simulink model "fiveleveldiode"  (Simulink 7.3)
settings: Solver=ode45  StartTime=0.0  StopTime=0.1  RelTol=1e-3
InitFcn:
  | clear;
  | clc;
  | f=50;
  | fs=4000;
libraries: powerlib x56, simulink x12, powerlib_extras x3
Description:
  | This model includes five level three phase diode clamped bridge. The control is implemented
  | using the multi carrier sinosoidal PWM technique.
  | 
  | This was created by Syed Abdul Rahman Kashif
  | University of Paderborn
  | Germany
settings Model: Creator=Kashif  LastModifiedBy=Sravani Harshini

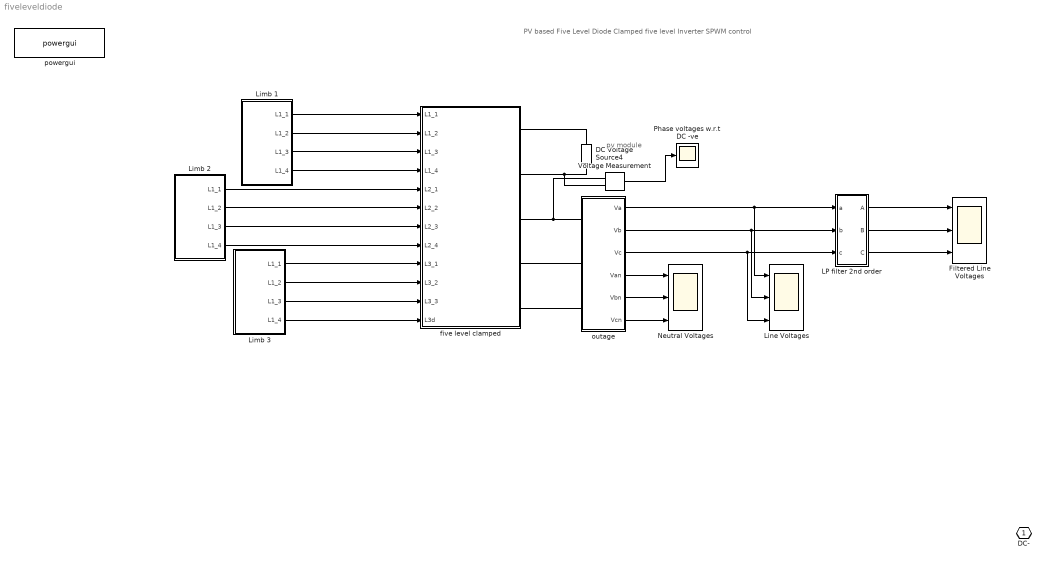
== system fiveleveldiode ==
  note: PV based Five Level Diode Clamped five level Inverter SPWM control
  note: pv module
  DC Voltage Source4 : powerlib/Electrical Sources/DC Voltage Source  DialogController=POWERSYS.PowerSysDialog  SystemSampleTime=-1  Amplitude=400  Measurements=None
  Filtered Line Voltages : Scope  NumInputPorts=3
      settings: YMin=-45~-35~-45  YMax=70~70~70  SaveName=Filtered_Line_Voltages  MaxDataPoints=5000000  SampleInput=on  SampleTime=5e-6
  LP filter 2nd order : Subsystem  mask{cutoff_frequency=500, damping_factor=0.707}
      mask prompts: cutoff_frequency "Cut off frequency"; damping_factor "Damping Factor"
  Limb 1 : Subsystem
  Limb 2 : Subsystem
  Limb 3 : Subsystem
  Line Voltages : Scope  NumInputPorts=3
      settings: YMin=-45~-35~-45  YMax=70~70~70  SaveName=Line_voltages  MaxDataPoints=5000000  SampleInput=on  SampleTime=5e-6
  Neutral Voltages : Scope  NumInputPorts=3
      settings: YMin=-45~-35~-45  YMax=70~70~70  SaveName=Neutral_voltages  MaxDataPoints=5000000  SampleInput=on  SampleTime=5e-6
  Phase voltages w.r.t DC -ve : Scope
      settings: YMin=0  YMax=100  SaveName=Phase_voltage_DC0  MaxDataPoints=5000000  SampleInput=on  SampleTime=5e-6
  Voltage Measurement : powerlib/Measurements/Voltage Measurement  DialogController=POWERSYS.PowerSysDialog  SystemSampleTime=-1  PhasorSimulation=off  OutputType=Complex  PSBequivalent=0
  five level clamped : Subsystem
      mask Description:
      | This includes five level three phase diode clamped bridge.
      | This was created by Syed Abdul Rahman Kashif
      | University of Paderborn
      | Germany
  outage : Subsystem
  powergui : powerlib/powergui  Priority=1  SystemSampleTime=-1  SimulationMode=Discrete  SampleTime=2e-6  frequency=60  SPID=off  DisableSnubberDevices=off  DisableRonSwitches=off  DisableVfSwitches=off  SwTol=0  Interpol=off  frequencyindice=0  echomessages=off  HookPort=off  DisplayEquations=off  FunctionMessages=off  EnableUseOfTLC=off  x0status=blocks  RestoreLinks=warning  Frange=[0:2:500]  Ylog=off  Xlog=on  ShowGrid=off  save=off  variable=ZData  structure=Filtered_Line_Voltages  ZoomFFT=off  StartTime=0.04  cycles=1  DisplayStyle=2  fundamental=50  FreqAxis=off  MaxFrequency=10000  frequencyindicesteady=1  RmsSteady=1  display=off  Ts=0  methode=off
  DC- : PMIOPort  Port=1  Side=Left
  wires:
  Limb 1/1(L1_1) -> five level clamped/1(L1_1)
  Limb 1/2(L1_2) -> five level clamped/2(L1_2)
  Limb 1/3(L1_3) -> five level clamped/3(L1_3)
  Limb 1/4(L1_4) -> five level clamped/4(L1_4)
  outage/4(Van) -> Neutral Voltages/1
  outage/5(Vbn) -> Neutral Voltages/2
  outage/6(Vcn) -> Neutral Voltages/3
  Voltage Measurement/1 -> Phase voltages w.r.t DC -ve/1
  Limb 2/1(L1_1) -> five level clamped/5(L2_1)
  Limb 2/2(L1_2) -> five level clamped/6(L2_2)
  Limb 2/3(L1_3) -> five level clamped/7(L2_3)
  Limb 2/4(L1_4) -> five level clamped/8(L2_4)
  Limb 3/1(L1_1) -> five level clamped/9(L3_1)
  Limb 3/2(L1_2) -> five level clamped/10(L3_2)
  Limb 3/3(L1_3) -> five level clamped/11(L3_3)
  Limb 3/4(L1_4) -> five level clamped/12(L3d)
  outage/1(Va) -> LP filter 2nd order/1(a), Line Voltages/1
  outage/2(Vb) -> LP filter 2nd order/2(b), Line Voltages/2
  outage/3(Vc) -> LP filter 2nd order/3(c), Line Voltages/3
  LP filter 2nd order/1(A) -> Filtered Line Voltages/1
  LP filter 2nd order/2(B) -> Filtered Line Voltages/2
  LP filter 2nd order/3(C) -> Filtered Line Voltages/3
  connections:
  five level clamped/RConn2 -- DC Voltage Source4/LConn1 -- Voltage Measurement/LConn2
  five level clamped/RConn1 -- DC Voltage Source4/RConn1
  five level clamped/RConn5 -- outage/LConn3
  five level clamped/RConn4 -- outage/LConn2
  five level clamped/RConn3 -- outage/LConn1 -- Voltage Measurement/LConn1

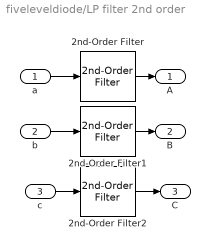
== system fiveleveldiode/LP filter 2nd order ==
  a : Inport  OutDataType=sfix(16)  OutScaling=2^0
  b : Inport  Port=2  OutDataType=sfix(16)  OutScaling=2^0
  c : Inport  Port=3  OutDataType=sfix(16)  OutScaling=2^0
  2nd-Order Filter : powerlib_extras/Control  Blocks/2nd-Order Filter  DialogController=POWERSYS.PowerSysDialog  SystemSampleTime=-1  FilterType=Lowpass  Fo=cutoff_frequency  Zeta=damping_factor  Initialize=off  Vac_Init=[1 45 60]  Vdc_Init=-0.5  PlotResponse=off  param1=[1 500 1]
  2nd-Order Filter1 : powerlib_extras/Control  Blocks/2nd-Order Filter  DialogController=POWERSYS.PowerSysDialog  SystemSampleTime=-1  FilterType=Lowpass  Fo=cutoff_frequency  Zeta=damping_factor  Initialize=off  Vac_Init=[1 45 60]  Vdc_Init=-0.5  PlotResponse=off  param1=[1 500 1]
  2nd-Order Filter2 : powerlib_extras/Control  Blocks/2nd-Order Filter  DialogController=POWERSYS.PowerSysDialog  SystemSampleTime=-1  FilterType=Lowpass  Fo=cutoff_frequency  Zeta=damping_factor  Initialize=off  Vac_Init=[1 45 60]  Vdc_Init=-0.5  PlotResponse=off  param1=[1 500 1]
  A : Outport  OutDataType=sfix(16)  OutScaling=2^0
  B : Outport  Port=2  OutDataType=sfix(16)  OutScaling=2^0
  C : Outport  Port=3  OutDataType=sfix(16)  OutScaling=2^0
  wires:
  a/1 -> 2nd-Order Filter/1
  2nd-Order Filter/1 -> A/1
  b/1 -> 2nd-Order Filter1/1
  2nd-Order Filter1/1 -> B/1
  c/1 -> 2nd-Order Filter2/1
  2nd-Order Filter2/1 -> C/1

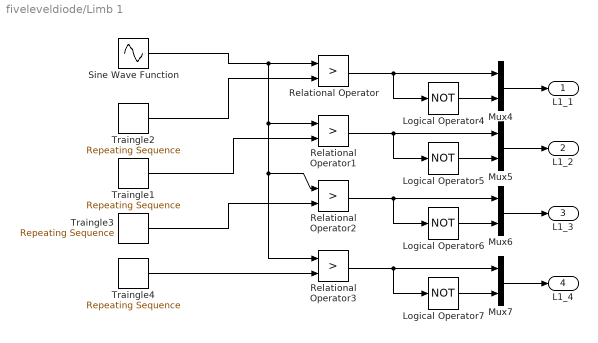
== system fiveleveldiode/Limb 1 ==
  Logical Operator{4..7} (4 alike) : Logic  Operator=NOT  AllPortsSameDT=off  OutDataTypeMode=boolean  OutDataTypeStr=boolean
  Mux{4..7} (4 alike) : Mux  Inputs=2
  Relational Operator{,1..3} (4 alike) : RelationalOperator  Operator=>  LogicOutDataTypeMode=boolean  LogicDataType=fixdt(0, 8)  OutDataTypeStr=boolean
  Sine Wave Function : Sin  Amplitude=5  Bias=5  Frequency=f*2*pi  Phase=0  Samples=10  SampleTime=0  Offset=0
  Traingle1 : simulink/Sources/Repeating Sequence  SystemSampleTime=-1  rep_seq_t=[0 1/fs]  rep_seq_y=[5 7.5]
  Traingle2 : simulink/Sources/Repeating Sequence  SystemSampleTime=-1  rep_seq_t=[0 1/fs]  rep_seq_y=[7.5 10]
  Traingle3 : simulink/Sources/Repeating Sequence  SystemSampleTime=-1  rep_seq_t=[0 1/fs]  rep_seq_y=[2.5 5]
  Traingle4 : simulink/Sources/Repeating Sequence  SystemSampleTime=-1  rep_seq_t=[0 1/fs]  rep_seq_y=[0 2.5]
  L1_1 : Outport  OutDataType=sfix(16)  OutScaling=2^0
  L1_2 : Outport  Port=2  OutDataType=sfix(16)  OutScaling=2^0
  L1_3 : Outport  Port=3  OutDataType=sfix(16)  OutScaling=2^0
  L1_4 : Outport  Port=4  OutDataType=sfix(16)  OutScaling=2^0
  wires:
  Sine Wave Function/1 -> Relational Operator/1, Relational Operator1/1, Relational Operator2/1, Relational Operator3/1
  Traingle2/1 -> Relational Operator/2
  Traingle4/1 -> Relational Operator3/2
  Traingle3/1 -> Relational Operator2/2
  Traingle1/1 -> Relational Operator1/2
  Relational Operator/1 -> Logical Operator4/1, Mux4/1
  Logical Operator4/1 -> Mux4/2
  Mux4/1 -> L1_1/1
  Relational Operator1/1 -> Mux5/1, Logical Operator5/1
  Logical Operator5/1 -> Mux5/2
  Mux5/1 -> L1_2/1
  Relational Operator2/1 -> Logical Operator6/1, Mux6/1
  Logical Operator6/1 -> Mux6/2
  Mux6/1 -> L1_3/1
  Relational Operator3/1 -> Mux7/1, Logical Operator7/1
  Logical Operator7/1 -> Mux7/2
  Mux7/1 -> L1_4/1

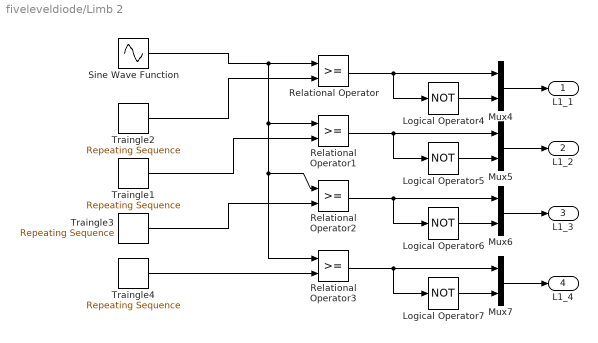
== system fiveleveldiode/Limb 2 ==
  Logical Operator{4..7} (4 alike) : Logic  Operator=NOT  AllPortsSameDT=off  OutDataTypeMode=boolean  OutDataTypeStr=boolean
  Mux{4..7} (4 alike) : Mux  Inputs=2
  Relational Operator{,1..3} (4 alike) : RelationalOperator  LogicOutDataTypeMode=boolean  LogicDataType=fixdt(0, 8)  OutDataTypeStr=boolean
  Sine Wave Function : Sin  Amplitude=5  Bias=5  Frequency=f*2*pi  Phase=4*pi/3  Samples=10  SampleTime=0  Offset=0
  Traingle1 : simulink/Sources/Repeating Sequence  SystemSampleTime=-1  rep_seq_t=[0 1/fs]  rep_seq_y=[5 7.5]
  Traingle2 : simulink/Sources/Repeating Sequence  SystemSampleTime=-1  rep_seq_t=[0 1/fs]  rep_seq_y=[7.5 10]
  Traingle3 : simulink/Sources/Repeating Sequence  SystemSampleTime=-1  rep_seq_t=[0 1/fs]  rep_seq_y=[2.5 5]
  Traingle4 : simulink/Sources/Repeating Sequence  SystemSampleTime=-1  rep_seq_t=[0 1/fs]  rep_seq_y=[0 2.5]
  L1_1 : Outport  OutDataType=sfix(16)  OutScaling=2^0
  L1_2 : Outport  Port=2  OutDataType=sfix(16)  OutScaling=2^0
  L1_3 : Outport  Port=3  OutDataType=sfix(16)  OutScaling=2^0
  L1_4 : Outport  Port=4  OutDataType=sfix(16)  OutScaling=2^0
  wires:
  Mux7/1 -> L1_4/1
  Logical Operator7/1 -> Mux7/2
  Relational Operator3/1 -> Logical Operator7/1, Mux7/1
  Mux6/1 -> L1_3/1
  Logical Operator6/1 -> Mux6/2
  Relational Operator2/1 -> Mux6/1, Logical Operator6/1
  Mux5/1 -> L1_2/1
  Logical Operator5/1 -> Mux5/2
  Relational Operator1/1 -> Logical Operator5/1, Mux5/1
  Mux4/1 -> L1_1/1
  Logical Operator4/1 -> Mux4/2
  Relational Operator/1 -> Mux4/1, Logical Operator4/1
  Traingle1/1 -> Relational Operator1/2
  Traingle3/1 -> Relational Operator2/2
  Traingle4/1 -> Relational Operator3/2
  Traingle2/1 -> Relational Operator/2
  Sine Wave Function/1 -> Relational Operator3/1, Relational Operator2/1, Relational Operator1/1, Relational Operator/1

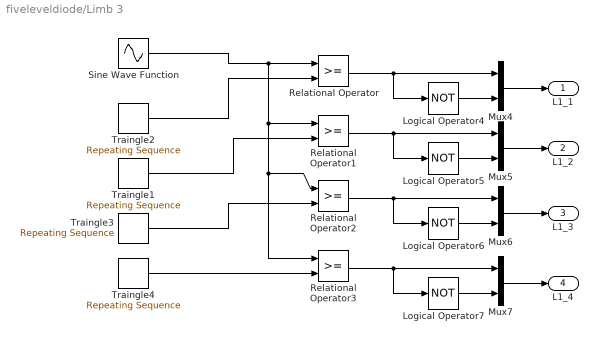
== system fiveleveldiode/Limb 3 ==
  Logical Operator{4..7} (4 alike) : Logic  Operator=NOT  AllPortsSameDT=off  OutDataTypeMode=boolean  OutDataTypeStr=boolean
  Mux{4..7} (4 alike) : Mux  Inputs=2
  Relational Operator{,1..3} (4 alike) : RelationalOperator  LogicOutDataTypeMode=boolean  LogicDataType=fixdt(0, 8)  OutDataTypeStr=boolean
  Sine Wave Function : Sin  Amplitude=5  Bias=5  Frequency=f*2*pi  Phase=2*pi/3  Samples=10  SampleTime=0  Offset=0
  Traingle1 : simulink/Sources/Repeating Sequence  SystemSampleTime=-1  rep_seq_t=[0 1/fs]  rep_seq_y=[5 7.5]
  Traingle2 : simulink/Sources/Repeating Sequence  SystemSampleTime=-1  rep_seq_t=[0 1/fs]  rep_seq_y=[7.5 10]
  Traingle3 : simulink/Sources/Repeating Sequence  SystemSampleTime=-1  rep_seq_t=[0 1/fs]  rep_seq_y=[2.5 5]
  Traingle4 : simulink/Sources/Repeating Sequence  SystemSampleTime=-1  rep_seq_t=[0 1/fs]  rep_seq_y=[0 2.5]
  L1_1 : Outport  OutDataType=sfix(16)  OutScaling=2^0
  L1_2 : Outport  Port=2  OutDataType=sfix(16)  OutScaling=2^0
  L1_3 : Outport  Port=3  OutDataType=sfix(16)  OutScaling=2^0
  L1_4 : Outport  Port=4  OutDataType=sfix(16)  OutScaling=2^0
  wires:
  Sine Wave Function/1 -> Relational Operator/1, Relational Operator1/1, Relational Operator2/1, Relational Operator3/1
  Traingle2/1 -> Relational Operator/2
  Traingle4/1 -> Relational Operator3/2
  Traingle3/1 -> Relational Operator2/2
  Traingle1/1 -> Relational Operator1/2
  Relational Operator/1 -> Logical Operator4/1, Mux4/1
  Logical Operator4/1 -> Mux4/2
  Mux4/1 -> L1_1/1
  Relational Operator1/1 -> Mux5/1, Logical Operator5/1
  Logical Operator5/1 -> Mux5/2
  Mux5/1 -> L1_2/1
  Relational Operator2/1 -> Logical Operator6/1, Mux6/1
  Logical Operator6/1 -> Mux6/2
  Mux6/1 -> L1_3/1
  Relational Operator3/1 -> Mux7/1, Logical Operator7/1
  Logical Operator7/1 -> Mux7/2
  Mux7/1 -> L1_4/1

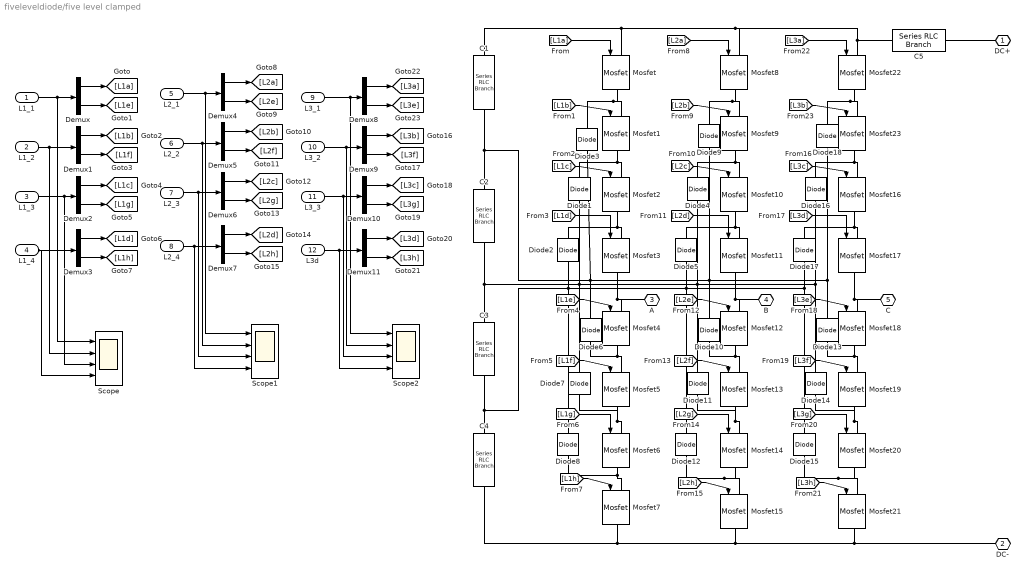
== system fiveleveldiode/five level clamped ==
  L1_1 : Inport  OutDataType=fixdt(1, 16)  OutScaling=2^0
  L1_2 : Inport  Port=2  OutDataType=fixdt(1, 16)  OutScaling=2^0
  L1_3 : Inport  Port=3  OutDataType=fixdt(1, 16)  OutScaling=2^0
  L1_4 : Inport  Port=4  OutDataType=fixdt(1, 16)  OutScaling=2^0
  L2_1 : Inport  Port=5  OutDataType=fixdt(1, 16)  OutScaling=2^0
  L2_2 : Inport  Port=6  OutDataType=fixdt(1, 16)  OutScaling=2^0
  L2_3 : Inport  Port=7  OutDataType=fixdt(1, 16)  OutScaling=2^0
  L2_4 : Inport  Port=8  OutDataType=fixdt(1, 16)  OutScaling=2^0
  L3_1 : Inport  Port=9  OutDataType=fixdt(1, 16)  OutScaling=2^0
  L3_2 : Inport  Port=10  OutDataType=fixdt(1, 16)  OutScaling=2^0
  L3_3 : Inport  Port=11  OutDataType=fixdt(1, 16)  OutScaling=2^0
  L3d : Inport  Port=12  OutDataType=fixdt(1, 16)  OutScaling=2^0
  C{1..4} (4 alike) : powerlib/Elements/Series RLC Branch  DialogController=POWERSYS.PowerSysDialog  PhysicalDomain=powersysdomain  SubClassName=unknown  LeftPortType=p1  RightPortType=p1  LConnTagsString=__new0  RConnTagsString=__new0  BranchType=C  Resistance=1  Inductance=1.0  SetiL0=off  InitialCurrent=0  Capacitance=2200e-6  Setx0=off  InitialVoltage=0  Measurements=None
  C5 : powerlib/Elements/Series RLC Branch  DialogController=POWERSYS.PowerSysDialog  PhysicalDomain=powersysdomain  SubClassName=unknown  LeftPortType=p1  RightPortType=p1  LConnTagsString=__new0  RConnTagsString=__new0  BranchType=R  Resistance=1  Inductance=1.0  SetiL0=off  InitialCurrent=0  Capacitance=2200e-6  Setx0=off  InitialVoltage=0  Measurements=None
  Demux{,1..11} (12 alike) : Demux  Outputs=2
  Diode{1..18} (18 alike) : powerlib/Power Electronics/Diode  DialogController=POWERSYS.PowerSysDialog  SystemSampleTime=-1  Ron=0.001  Lon=0  Vf=0.8  IC=0  UseSnubber=off  Rs=500  Cs=250e-9  Measurements=off
  Mosfet{,1..23} (24 alike) : powerlib/Power Electronics/Mosfet  DialogController=POWERSYS.PowerSysDialog  SystemSampleTime=-1  Ron=0.1  Lon=0  Rd=0.01  Vfd=0  IC=0  Rs=1e5  Cs=inf  Measurements=off
  Scope : Scope  NumInputPorts=4
      settings: YMin=-5~-5~-5~-5  YMax=5~5~5~5  MaxDataPoints=5000000
  Scope1 : Scope  NumInputPorts=4
      settings: YMin=-5~-5~-5~-5  YMax=5~5~5~5  SaveName=ScopeData2  MaxDataPoints=5000000
  Scope2 : Scope  NumInputPorts=4
      settings: YMin=-5~-5~-5~-5  YMax=5~5~5~5  SaveName=ScopeData3  MaxDataPoints=5000000
  DC+ : PMIOPort  Port=1  Side=Right
  DC- : PMIOPort  Port=2  Side=Right
  A : PMIOPort  Port=3  Side=Right
  B : PMIOPort  Port=4  Side=Right
  C : PMIOPort  Port=5  Side=Right
  wires:
  Demux/1 -> [L1a]
  Demux/2 -> [L1e]
  Demux1/1 -> [L1b]
  Demux1/2 -> [L1f]
  Demux2/1 -> [L1c]
  Demux2/2 -> [L1g]
  Demux3/1 -> [L1d]
  Demux3/2 -> [L1h]
  L1_1/1 -> Demux/1, Scope/1
  L1_2/1 -> Demux1/1, Scope/2
  L1_3/1 -> Demux2/1, Scope/3
  L1_4/1 -> Demux3/1, Scope/4
  Demux4/1 -> [L2a]
  Demux4/2 -> [L2e]
  Demux5/1 -> [L2b]
  Demux5/2 -> [L2f]
  Demux6/1 -> [L2c]
  Demux6/2 -> [L2g]
  Demux7/1 -> [L2d]
  Demux7/2 -> [L2h]
  L2_1/1 -> Demux4/1, Scope1/1
  L2_2/1 -> Demux5/1, Scope1/2
  L2_3/1 -> Demux6/1, Scope1/3
  L2_4/1 -> Demux7/1, Scope1/4
  Demux8/1 -> [L3a]
  Demux8/2 -> [L3e]
  Demux9/1 -> [L3b]
  Demux9/2 -> [L3f]
  Demux10/1 -> [L3c]
  Demux10/2 -> [L3g]
  Demux11/1 -> [L3d]
  Demux11/2 -> [L3h]
  L3_1/1 -> Demux8/1, Scope2/1
  L3_2/1 -> Demux9/1, Scope2/2
  L3_3/1 -> Demux10/1, Scope2/3
  L3d/1 -> Demux11/1, Scope2/4
  [L1a] -> Mosfet/1
  [L1b] -> Mosfet1/1
  [L1c] -> Mosfet2/1
  [L1d] -> Mosfet3/1
  [L1e] -> Mosfet4/1
  [L1f] -> Mosfet5/1
  [L1g] -> Mosfet6/1
  [L1h] -> Mosfet7/1
  [L2a] -> Mosfet8/1
  [L2b] -> Mosfet9/1
  [L2c] -> Mosfet10/1
  [L2d] -> Mosfet11/1
  [L2e] -> Mosfet12/1
  [L2f] -> Mosfet13/1
  [L2g] -> Mosfet14/1
  [L2h] -> Mosfet15/1
  [L3a] -> Mosfet22/1
  [L3b] -> Mosfet23/1
  [L3c] -> Mosfet16/1
  [L3d] -> Mosfet17/1
  [L3e] -> Mosfet18/1
  [L3f] -> Mosfet19/1
  [L3g] -> Mosfet20/1
  [L3h] -> Mosfet21/1
  connections:
  Diode3/RConn1 -- Mosfet1/LConn1 -- Mosfet/RConn1
  Mosfet1/RConn1 -- Mosfet2/LConn1 -- Diode1/RConn1
  Mosfet3/RConn1 -- Mosfet4/LConn1 -- A/RConn1
  Diode2/RConn1 -- Mosfet2/RConn1 -- Mosfet3/LConn1
  Diode6/LConn1 -- Mosfet4/RConn1 -- Mosfet5/LConn1
  Mosfet5/RConn1 -- Mosfet6/LConn1 -- Diode7/LConn1
  Diode9/RConn1 -- Mosfet8/RConn1 -- Mosfet9/LConn1
  Mosfet9/RConn1 -- Diode4/RConn1 -- Mosfet10/LConn1
  Mosfet11/RConn1 -- B/RConn1 -- Mosfet12/LConn1
  Diode5/RConn1 -- Mosfet11/LConn1 -- Mosfet10/RConn1
  Diode10/LConn1 -- Mosfet13/LConn1 -- Mosfet12/RConn1
  Mosfet13/RConn1 -- Diode11/LConn1 -- Mosfet14/LConn1
  Mosfet14/RConn1 -- Diode12/LConn1 -- Mosfet15/LConn1
  Diode1/LConn1 -- Diode7/RConn1 -- Diode4/LConn1 -- Diode11/RConn1 -- Diode14/RConn1 -- Diode16/LConn1 -- C2/RConn1 -- C3/LConn1
  Mosfet22/RConn1 -- Mosfet23/LConn1 -- Diode18/RConn1
  Diode16/RConn1 -- Mosfet16/LConn1 -- Mosfet23/RConn1
  C/RConn1 -- Mosfet18/LConn1 -- Mosfet17/RConn1
  Mosfet17/LConn1 -- Mosfet16/RConn1 -- Diode17/RConn1
  Mosfet19/LConn1 -- Mosfet18/RConn1 -- Diode13/LConn1
  Diode14/LConn1 -- Mosfet20/LConn1 -- Mosfet19/RConn1
  Mosfet20/RConn1 -- Diode15/LConn1 -- Mosfet21/LConn1
  Mosfet22/LConn1 -- Mosfet8/LConn1 -- Mosfet/LConn1 -- C1/LConn1 -- C5/LConn1
  Mosfet7/RConn1 -- Mosfet15/RConn1 -- Mosfet21/RConn1 -- DC-/RConn1 -- C4/RConn1
  C1/RConn1 -- C2/LConn1 -- Diode3/LConn1 -- Diode6/RConn1 -- Diode9/LConn1 -- Diode10/RConn1 -- Diode13/RConn1 -- Diode18/LConn1
  C3/RConn1 -- C4/LConn1 -- Diode2/LConn1 -- Diode8/RConn1 -- Diode5/LConn1 -- Diode12/RConn1 -- Diode15/RConn1 -- Diode17/LConn1
  C5/RConn1 -- DC+/RConn1
  Mosfet6/RConn1 -- Mosfet7/LConn1 -- Diode8/LConn1

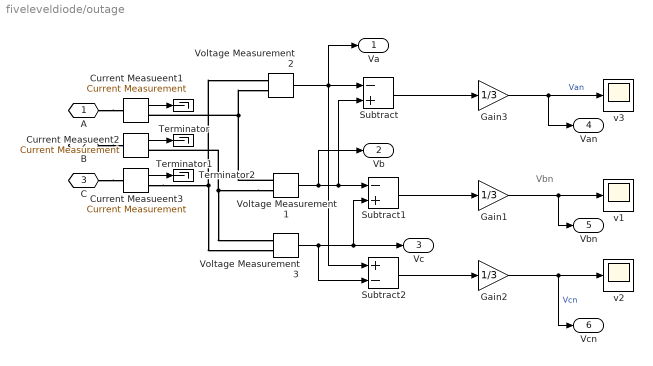
== system fiveleveldiode/outage ==
  note: Vbn
  Current Measueent1 : powerlib/Measurements/Current Measurement  DialogController=POWERSYS.PowerSysDialog  SystemSampleTime=-1  PhasorSimulation=off  OutputType=Complex  PSBequivalent=0
  Current Measueent2 : powerlib/Measurements/Current Measurement  DialogController=POWERSYS.PowerSysDialog  SystemSampleTime=-1  PhasorSimulation=off  OutputType=Complex  PSBequivalent=0
  Current Measueent3 : powerlib/Measurements/Current Measurement  DialogController=POWERSYS.PowerSysDialog  SystemSampleTime=-1  PhasorSimulation=off  OutputType=Complex  PSBequivalent=0
  Gain1 : Gain  Gain=1/3  ParameterDataType=sfix(16)  ParameterScaling=2^0  OutDataType=sfix(16)  OutScaling=2^0
  Gain2 : Gain  Gain=1/3  ParameterDataType=sfix(16)  ParameterScaling=2^0  OutDataType=sfix(16)  OutScaling=2^0
  Gain3 : Gain  Gain=1/3  ParameterDataType=sfix(16)  ParameterScaling=2^0  OutDataType=sfix(16)  OutScaling=2^0
  Subtract : Sum  Inputs=-+  OutDataType=sfix(16)  OutScaling=2^-10
  Subtract1 : Sum  Inputs=-+  OutDataType=sfix(16)  OutScaling=2^-10
  Subtract2 : Sum  Inputs=+-  OutDataType=sfix(16)  OutScaling=2^-10
  Terminator : Terminator
  Terminator1 : Terminator
  Terminator2 : Terminator
  Voltage Measurement1 : powerlib/Measurements/Voltage Measurement  DialogController=POWERSYS.PowerSysDialog  SystemSampleTime=-1  PhasorSimulation=off  OutputType=Complex  PSBequivalent=0
  Voltage Measurement2 : powerlib/Measurements/Voltage Measurement  DialogController=POWERSYS.PowerSysDialog  SystemSampleTime=-1  PhasorSimulation=off  OutputType=Complex  PSBequivalent=0
  Voltage Measurement3 : powerlib/Measurements/Voltage Measurement  DialogController=POWERSYS.PowerSysDialog  SystemSampleTime=-1  PhasorSimulation=off  OutputType=Complex  PSBequivalent=0
  v1 : Scope
      settings: SaveName=ScopeData25  MaxDataPoints=5000000
  v2 : Scope
      settings: SaveName=ScopeData26  MaxDataPoints=5000000
  v3 : Scope
      settings: YMin=-300  YMax=300  SaveName=ScopeData27  MaxDataPoints=5000000
  A : PMIOPort  Port=1  Side=Left
  B : PMIOPort  Port=2  Side=Left
  C : PMIOPort  Port=3  Side=Left
  Va : Outport  OutDataType=sfix(16)  OutScaling=2^0
  Vb : Outport  Port=2  OutDataType=sfix(16)  OutScaling=2^0
  Vc : Outport  Port=3  OutDataType=sfix(16)  OutScaling=2^0
  Van : Outport  Port=4  OutDataType=sfix(16)  OutScaling=2^0
  Vbn : Outport  Port=5  OutDataType=sfix(16)  OutScaling=2^0
  Vcn : Outport  Port=6  OutDataType=sfix(16)  OutScaling=2^0
  wires:
  Gain2/1 -> v2/1, Vcn/1  "Vcn"
  Subtract2/1 -> Gain2/1
  Gain1/1 -> v1/1, Vbn/1
  Subtract1/1 -> Gain1/1
  Voltage Measurement3/1 -> Subtract2/2, Subtract1/2, Vc/1
  Gain3/1 -> v3/1, Van/1  "Van"
  Subtract/1 -> Gain3/1
  Voltage Measurement1/1 -> Subtract/2, Subtract1/1, Vb/1
  Voltage Measurement2/1 -> Subtract/1, Subtract2/1, Va/1
  Current Measueent1/1 -> Terminator/1
  Current Measueent2/1 -> Terminator1/1
  Current Measueent3/1 -> Terminator2/1
  connections:
  Voltage Measurement1/LConn1 -- Current Measueent1/RConn1 -- Voltage Measurement2/LConn2
  Voltage Measurement1/LConn2 -- Current Measueent2/RConn1 -- Voltage Measurement3/LConn1
  Current Measueent3/RConn1 -- Voltage Measurement2/LConn1 -- Voltage Measurement3/LConn2
  A/RConn1 -- Current Measueent1/LConn1
  B/RConn1 -- Current Measueent2/LConn1
  C/RConn1 -- Current Measueent3/LConn1
